simulink model "janrit"  (R2026a)
settings: Solver=ode45  StopTime=6
values from neighbouring files (symbols this model uses):
  A = 7    [wencode.m]
  B = 15    [wencode.m]
undefined symbols (not defined in the file or in its folder): a, b, C1
libraries: simulink x1
settings Model: Creator=acer  LastModifiedBy=acer

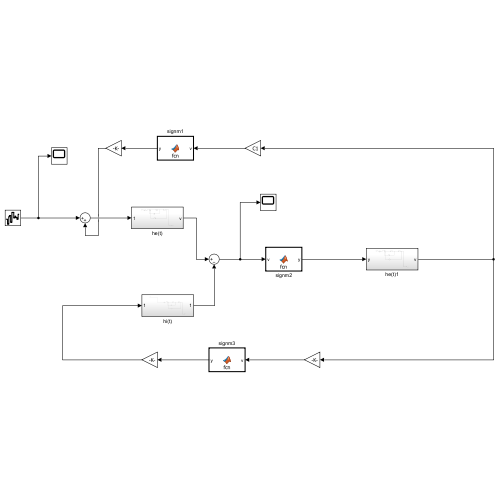
[thumbnail: Simulink's stored preview of the top-level diagram]
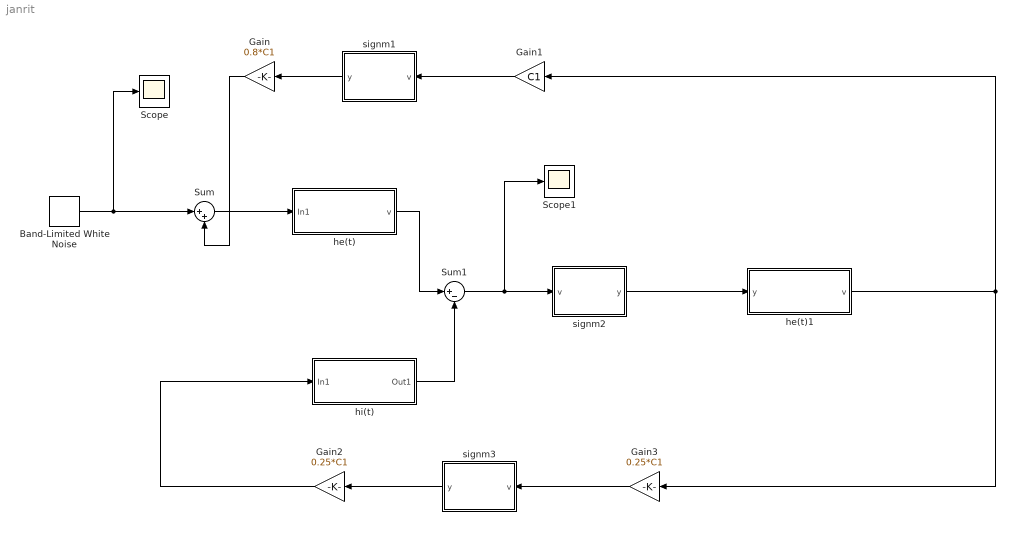
== system janrit ==
  Band-Limited White Noise : simulink/Sources/Band-Limited White Noise  Cov=[1]  Ts=0.001  seed=[23341]
  Gain : Gain  Gain=0.8*C1
  Gain1 : Gain  Gain=C1
  Gain2 : Gain  Gain=0.25*C1
  Gain3 : Gain  Gain=0.25*C1
  Scope : Scope
      settings: ActiveDisplayYMinimum=-1  ActiveDisplayYMaximum=1
  Scope1 : Scope
      settings: ActiveDisplayYMinimum=-12.018339812364449  ActiveDisplayYMaximum=24.128278137585305
  Sum : Sum  Inputs=|++
  Sum1 : Sum  Inputs=|+-
  he(t) : Subsystem
  he(t)1 : Subsystem
  hi(t) : Subsystem
  signm1 : MATLAB Function  TreatAsAtomicUnit=on
  signm2 : MATLAB Function  TreatAsAtomicUnit=on
  signm3 : MATLAB Function  TreatAsAtomicUnit=on
  wires:
  Band-Limited White Noise/1 -> Scope/1, Sum/1
  Sum/1 -> he(t)/1(In1)
  he(t)/1(v) -> Sum1/1
  Sum1/1 -> Scope1/1, signm2/1(v)
  signm2/1(y) -> he(t)1/1(y)
  hi(t)/1(Out1) -> Sum1/2
  Gain2/1 -> hi(t)/1(In1)
  signm3/1(y) -> Gain2/1
  Gain3/1 -> signm3/1(v)
  signm1/1(y) -> Gain/1
  Gain1/1 -> signm1/1(v)
  he(t)1/1(v) -> Gain1/1, Gain3/1
  Gain/1 -> Sum/2

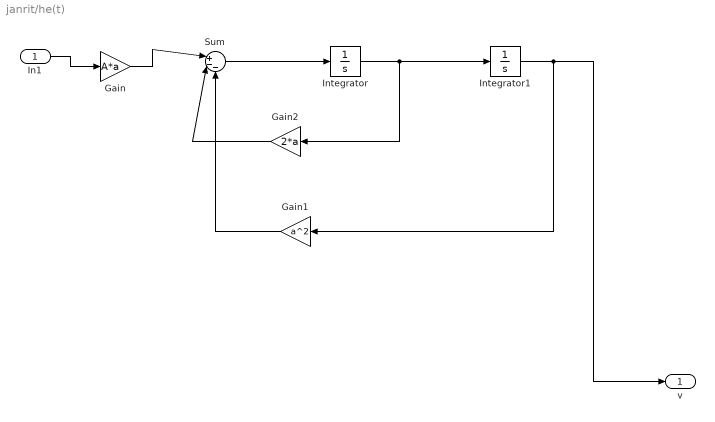
== system janrit/he(t) ==
  In1 : Inport
  Gain : Gain  Gain=A*a
  Gain1 : Gain  Gain=a^2
  Gain2 : Gain  Gain=2*a
  Integrator : Integrator
  Integrator1 : Integrator
  Sum : Sum  Inputs=|+--
  v : Outport
  wires:
  In1/1 -> Gain/1
  Gain/1 -> Sum/1
  Sum/1 -> Integrator/1
  Integrator/1 -> Gain2/1, Integrator1/1
  Integrator1/1 -> Gain1/1, v/1
  Gain2/1 -> Sum/2
  Gain1/1 -> Sum/3

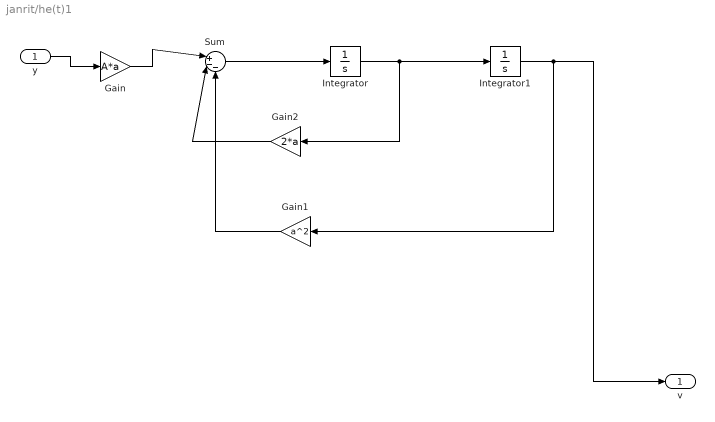
== system janrit/he(t)1 ==
  y : Inport
  Gain : Gain  Gain=A*a
  Gain1 : Gain  Gain=a^2
  Gain2 : Gain  Gain=2*a
  Integrator : Integrator
  Integrator1 : Integrator
  Sum : Sum  Inputs=|+--
  v : Outport
  wires:
  y/1 -> Gain/1
  Gain/1 -> Sum/1
  Sum/1 -> Integrator/1
  Integrator/1 -> Gain2/1, Integrator1/1
  Integrator1/1 -> Gain1/1, v/1
  Gain2/1 -> Sum/2
  Gain1/1 -> Sum/3

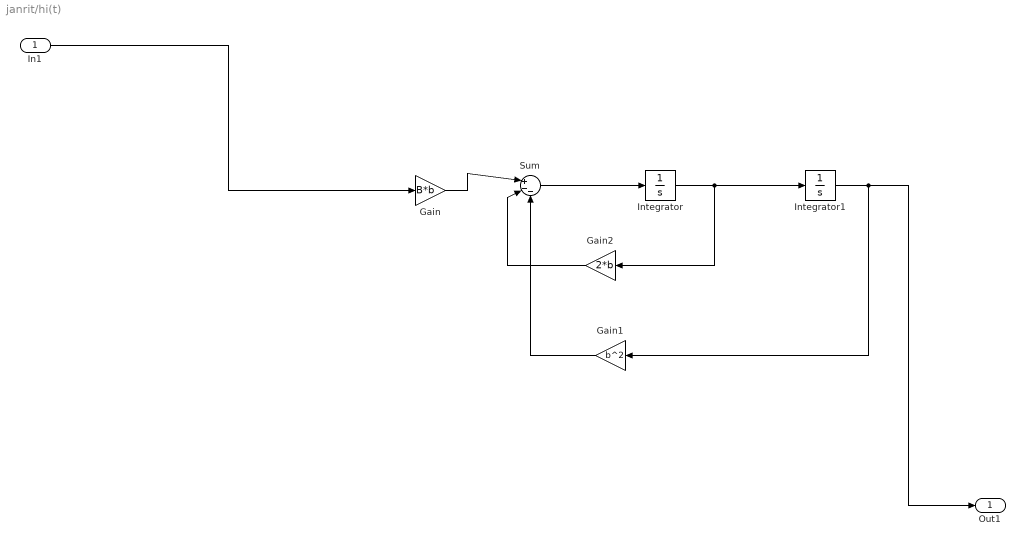
== system janrit/hi(t) ==
  In1 : Inport
  Gain : Gain  Gain=B*b
  Gain1 : Gain  Gain=b^2
  Gain2 : Gain  Gain=2*b
  Integrator : Integrator
  Integrator1 : Integrator
  Sum : Sum  Inputs=|+--
  Out1 : Outport
  wires:
  Integrator/1 -> Integrator1/1, Gain2/1
  Gain/1 -> Sum/1
  Integrator1/1 -> Out1/1, Gain1/1
  Sum/1 -> Integrator/1
  Gain2/1 -> Sum/2
  Gain1/1 -> Sum/3
  In1/1 -> Gain/1

== matlab function janrit/signm1 ==
  data: v input; y output
function y=fcn(v)

e0=2.5;
v0=6;
r=0.56;

y=(2*e0)/(1+exp(r*(v0-v)));

end

== matlab function janrit/signm3 ==
  data: v input; y output
function y=fcn(v)

e0=2.5;
v0=6;
r=0.56;

y=(2*e0)/(1+exp(r*(v0-v)));

end

== matlab function janrit/signm2 ==
  data: v input; y output
function y=fcn(v)

e0=2.5;
v0=6;
r=0.56;

y=(2*e0)/(1+exp(r*(v0-v)));

end
